simulink model "test_mdl_NI"  (R2018a)
settings: Solver=VariableStepAuto  StartTime=0.0  StopTime=10.0  RelTol=1e-3
(part 14 of 24)

== system test_mdl_NI/Subsystem/SOBDMC_HPCM_FD1/GoTimeSettings_FD1_Ox3F8 ==
  in_port : Inport
  ChrgGoTAllOn_B_Stat : Terminator
  ChrgGoTElement_B_Dsply : Terminator
  ChrgGoTElement_D_Stat : Terminator
  ChrgGoTExtHtrEnbl_B_Rq : Terminator
  ChrgGoTExtHtr_B_Stat : Terminator
  ChrgGoTHr_T_Stat : Terminator
  ChrgGoTMnte_D_Stat : Terminator
  ChrgGoTNext_D_Stat : Terminator
  ChrgGoTPrcond_D_Stat : Terminator
  ChrgGoTTouchEnbl_B_Rq : Terminator
  ChrgGoTTouch_B_Stat : Terminator
  ChrgLocIdCurnt_D_Uns : Terminator
  bus_selector : BusSelector  OutputSignals=ChrgGoTAllOn_B_Stat,ChrgGoTElement_B_Dsply,ChrgGoTElement_D_Stat,ChrgGoTExtHtrEnbl_B_Rq,ChrgGoTExtHtr_B_Stat,ChrgGoTHr_T_Stat,ChrgGoTMnte_D_Stat,ChrgGoTNext_D_Stat,ChrgGoTPrcond_D_Stat,ChrgGoTTouchEnbl_B_Rq,ChrgGoTTouch_B_Stat,ChrgLocIdCurnt_D_Uns
  wires:
  in_port/1 -> bus_selector/1  "GoTimeSettings_FD1_Ox3F8"
  bus_selector/1 -> ChrgGoTAllOn_B_Stat/1  "<ChrgGoTAllOn_B_Stat>"
  bus_selector/2 -> ChrgGoTElement_B_Dsply/1  "<ChrgGoTElement_B_Dsply>"
  bus_selector/3 -> ChrgGoTElement_D_Stat/1  "<ChrgGoTElement_D_Stat>"
  bus_selector/4 -> ChrgGoTExtHtrEnbl_B_Rq/1  "<ChrgGoTExtHtrEnbl_B_Rq>"
  bus_selector/5 -> ChrgGoTExtHtr_B_Stat/1  "<ChrgGoTExtHtr_B_Stat>"
  bus_selector/6 -> ChrgGoTHr_T_Stat/1  "<ChrgGoTHr_T_Stat>"
  bus_selector/7 -> ChrgGoTMnte_D_Stat/1  "<ChrgGoTMnte_D_Stat>"
  bus_selector/8 -> ChrgGoTNext_D_Stat/1  "<ChrgGoTNext_D_Stat>"
  bus_selector/9 -> ChrgGoTPrcond_D_Stat/1  "<ChrgGoTPrcond_D_Stat>"
  bus_selector/10 -> ChrgGoTTouchEnbl_B_Rq/1  "<ChrgGoTTouchEnbl_B_Rq>"
  bus_selector/11 -> ChrgGoTTouch_B_Stat/1  "<ChrgGoTTouch_B_Stat>"
  bus_selector/12 -> ChrgLocIdCurnt_D_Uns/1  "<ChrgLocIdCurnt_D_Uns>"

== system test_mdl_NI/Subsystem/SOBDMC_HPCM_FD1/HEV_ChargeStat_FD1_Ox352 ==
  in_port : Inport
  ChargeNowDuration_St : Terminator
  EstmChrgTimeHP_St : Terminator
  EstmChrgTimeLP_St : Terminator
  NxtUsgSocEst_Pc_Dsply : Terminator
  VehElRngeNut_L_Dsply : Terminator
  bus_selector : BusSelector  OutputSignals=ChargeNowDuration_St,EstmChrgTimeHP_St,EstmChrgTimeLP_St,NxtUsgSocEst_Pc_Dsply,VehElRngeNut_L_Dsply
  wires:
  in_port/1 -> bus_selector/1  "HEV_ChargeStat_FD1_Ox352"
  bus_selector/1 -> ChargeNowDuration_St/1  "<ChargeNowDuration_St>"
  bus_selector/2 -> EstmChrgTimeHP_St/1  "<EstmChrgTimeHP_St>"
  bus_selector/3 -> EstmChrgTimeLP_St/1  "<EstmChrgTimeLP_St>"
  bus_selector/4 -> NxtUsgSocEst_Pc_Dsply/1  "<NxtUsgSocEst_Pc_Dsply>"
  bus_selector/5 -> VehElRngeNut_L_Dsply/1  "<VehElRngeNut_L_Dsply>"

== system test_mdl_NI/Subsystem/SOBDMC_HPCM_FD1/MHT_EV_Wakeup_FD1_Ox478 ==
  in_port : Inport
  BattChlrSov_B_Rq : Terminator
  BattChrgTrgtSoC_D_Rq : Terminator
  BattTracClntVlv_B_Rq : Terminator
  BattTracDrvSustn_B_Rq : Terminator
  BrkAppl_D_RqPt : Terminator
  CabinDrvSustn_B_Rq : Terminator
  CabnEvapSovFront_B_Rq : Terminator
  CabnEvapSovRear_B_Rq : Terminator
  ChrgNowEvnt_B_Stat : Terminator
  HeatCoreSovRear_B_Rq : Terminator
  HtrnClntFlw_D_Rq : Terminator
  HtrnCnnctPwr_B_Stat : Terminator
  HtrnDcdcDis_B_Rq : Terminator
  PreCondBatt_B_Actl : Terminator
  PtcHtr_D_Stat : Terminator
  WakeAlarm0_B_Typ : Terminator
  WakeAlarm0_T_Rq : Terminator
  bus_selector : BusSelector  OutputSignals=BattChlrSov_B_Rq,BattChrgTrgtSoC_D_Rq,BattTracClntVlv_B_Rq,BattTracDrvSustn_B_Rq,BrkAppl_D_RqPt,CabinDrvSustn_B_Rq,CabnEvapSovFront_B_Rq,CabnEvapSovRear_B_Rq,ChrgNowEvnt_B_Stat,HeatCoreSovRear_B_Rq,HtrnClntFlw_D_Rq,HtrnCnnctPwr_B_Stat,HtrnDcdcDis_B_Rq,PreCondBatt_B_Actl,PtcHtr_D_Stat,WakeAlarm0_B_Typ,WakeAlarm0_T_Rq
  wires:
  in_port/1 -> bus_selector/1  "MHT_EV_Wakeup_FD1_Ox478"
  bus_selector/1 -> BattChlrSov_B_Rq/1  "<BattChlrSov_B_Rq>"
  bus_selector/2 -> BattChrgTrgtSoC_D_Rq/1  "<BattChrgTrgtSoC_D_Rq>"
  bus_selector/3 -> BattTracClntVlv_B_Rq/1  "<BattTracClntVlv_B_Rq>"
  bus_selector/4 -> BattTracDrvSustn_B_Rq/1  "<BattTracDrvSustn_B_Rq>"
  bus_selector/5 -> BrkAppl_D_RqPt/1  "<BrkAppl_D_RqPt>"
  bus_selector/6 -> CabinDrvSustn_B_Rq/1  "<CabinDrvSustn_B_Rq>"
  bus_selector/7 -> CabnEvapSovFront_B_Rq/1  "<CabnEvapSovFront_B_Rq>"
  bus_selector/8 -> CabnEvapSovRear_B_Rq/1  "<CabnEvapSovRear_B_Rq>"
  bus_selector/9 -> ChrgNowEvnt_B_Stat/1  "<ChrgNowEvnt_B_Stat>"
  bus_selector/10 -> HeatCoreSovRear_B_Rq/1  "<HeatCoreSovRear_B_Rq>"
  bus_selector/11 -> HtrnClntFlw_D_Rq/1  "<HtrnClntFlw_D_Rq>"
  bus_selector/12 -> HtrnCnnctPwr_B_Stat/1  "<HtrnCnnctPwr_B_Stat>"
  bus_selector/13 -> HtrnDcdcDis_B_Rq/1  "<HtrnDcdcDis_B_Rq>"
  bus_selector/14 -> PreCondBatt_B_Actl/1  "<PreCondBatt_B_Actl>"
  bus_selector/15 -> PtcHtr_D_Stat/1  "<PtcHtr_D_Stat>"
  bus_selector/16 -> WakeAlarm0_B_Typ/1  "<WakeAlarm0_B_Typ>"
  bus_selector/17 -> WakeAlarm0_T_Rq/1  "<WakeAlarm0_T_Rq>"

== system test_mdl_NI/Subsystem/SOBDMC_HPCM_FD1/MtrTracData_1_FD1_Ox441 ==
  in_port : Inport
  Inv1_Te_Actl : Terminator
  Mtr2Aout_W_ActlMntr : Terminator
  Mtr2CntlTeAlrm_B_Stat : Terminator
  MtrTrac2Coil_Te_Actl : Terminator
  MtrTrac2Falt_B_Stat : Terminator
  MtrTrac2Inv_Te_Actl : Terminator
  MtrTrac2TeAlrm_B_Stat : Terminator
  MtrTrac2_I_Actl : Terminator
  MtrTrac2_U_Actl : Terminator
  bus_selector : BusSelector  OutputSignals=Inv1_Te_Actl,Mtr2Aout_W_ActlMntr,Mtr2CntlTeAlrm_B_Stat,MtrTrac2Coil_Te_Actl,MtrTrac2Falt_B_Stat,MtrTrac2Inv_Te_Actl,MtrTrac2TeAlrm_B_Stat,MtrTrac2_I_Actl,MtrTrac2_U_Actl
  wires:
  in_port/1 -> bus_selector/1  "MtrTracData_1_FD1_Ox441"
  bus_selector/1 -> Inv1_Te_Actl/1  "<Inv1_Te_Actl>"
  bus_selector/2 -> Mtr2Aout_W_ActlMntr/1  "<Mtr2Aout_W_ActlMntr>"
  bus_selector/3 -> Mtr2CntlTeAlrm_B_Stat/1  "<Mtr2CntlTeAlrm_B_Stat>"
  bus_selector/4 -> MtrTrac2Coil_Te_Actl/1  "<MtrTrac2Coil_Te_Actl>"
  bus_selector/5 -> MtrTrac2Falt_B_Stat/1  "<MtrTrac2Falt_B_Stat>"
  bus_selector/6 -> MtrTrac2Inv_Te_Actl/1  "<MtrTrac2Inv_Te_Actl>"
  bus_selector/7 -> MtrTrac2TeAlrm_B_Stat/1  "<MtrTrac2TeAlrm_B_Stat>"
  bus_selector/8 -> MtrTrac2_I_Actl/1  "<MtrTrac2_I_Actl>"
  bus_selector/9 -> MtrTrac2_U_Actl/1  "<MtrTrac2_U_Actl>"

== system test_mdl_NI/Subsystem/SOBDMC_HPCM_FD1/MtrTrac_Data2_FD1_Ox442 ==
  in_port : Inport
  ChrgStat_D_ActlMntr : Terminator
  HybVehMde_D_ActlMntr : Terminator
  Inv1Ain_I_ActlMntr : Terminator
  Mtr2State_D_ActlMntr : Terminator
  VehElRnge_L_Dsply : Terminator
  bus_selector : BusSelector  OutputSignals=ChrgStat_D_ActlMntr,HybVehMde_D_ActlMntr,Inv1Ain_I_ActlMntr,Mtr2State_D_ActlMntr,VehElRnge_L_Dsply
  wires:
  in_port/1 -> bus_selector/1  "MtrTrac_Data2_FD1_Ox442"
  bus_selector/1 -> ChrgStat_D_ActlMntr/1  "<ChrgStat_D_ActlMntr>"
  bus_selector/2 -> HybVehMde_D_ActlMntr/1  "<HybVehMde_D_ActlMntr>"
  bus_selector/3 -> Inv1Ain_I_ActlMntr/1  "<Inv1Ain_I_ActlMntr>"
  bus_selector/4 -> Mtr2State_D_ActlMntr/1  "<Mtr2State_D_ActlMntr>"
  bus_selector/5 -> VehElRnge_L_Dsply/1  "<VehElRnge_L_Dsply>"

== system test_mdl_NI/Subsystem/SOBDMC_HPCM_FD1/OTAPhysSOBDMCtoGWM_FD1_Ox1B936011 ==
  in_port : Inport
  OTAPhysHPCMtoGWM_ECG : Terminator
  bus_selector : BusSelector  OutputSignals=OTAPhysHPCMtoGWM_ECG
  wires:
  in_port/1 -> bus_selector/1  "OTAPhysSOBDMCtoGWM_FD1_Ox1B936011"
  bus_selector/1 -> OTAPhysHPCMtoGWM_ECG/1  "<OTAPhysHPCMtoGWM_ECG>"

== system test_mdl_NI/Subsystem/SOBDMC_HPCM_FD1/PARSEDHPCMtoGWM_ECG_FD1_Ox1BA36011 ==
  in_port : Inport
  PARSEDPhysHPCMtoGWM_ECG : Terminator
  bus_selector : BusSelector  OutputSignals=PARSEDPhysHPCMtoGWM_ECG
  wires:
  in_port/1 -> bus_selector/1  "PARSEDHPCMtoGWM_ECG_FD1_Ox1BA36011"
  bus_selector/1 -> PARSEDPhysHPCMtoGWM_ECG/1  "<PARSEDPhysHPCMtoGWM_ECG>"

== system test_mdl_NI/Subsystem/SOBDMC_HPCM_FD1/PARSEDPushSOBDMCtoGWM_FD1_Ox1BB36011 ==
  in_port : Inport
  PARSEDPhysHPCM2toGWM_ECG : Terminator
  bus_selector : BusSelector  OutputSignals=PARSEDPhysHPCM2toGWM_ECG
  wires:
  in_port/1 -> bus_selector/1  "PARSEDPushSOBDMCtoGWM_FD1_Ox1BB36011"
  bus_selector/1 -> PARSEDPhysHPCM2toGWM_ECG/1  "<PARSEDPhysHPCM2toGWM_ECG>"

== system test_mdl_NI/Subsystem/SOBDMC_HPCM_FD1/PreCond_Hev_Data1_FD1_Ox440 ==
  in_port : Inport
  BattChrgInhbt_D_Rq : Terminator
  ChrgStat_D2_Dsply : Terminator
  ChrgTMatch_B_Stat : Terminator
  HvacPrecondAC_D_Rq : Terminator
  HvacPrecondBlwr2_D_Rq : Terminator
  HvacPrecondMode2_D_Rq : Terminator
  HvacPrecondRecirc_D_Rq : Terminator
  HvacPrecond_Te_Rq : Terminator
  bus_selector : BusSelector  OutputSignals=BattChrgInhbt_D_Rq,ChrgStat_D2_Dsply,ChrgTMatch_B_Stat,HvacPrecondAC_D_Rq,HvacPrecondBlwr2_D_Rq,HvacPrecondMode2_D_Rq,HvacPrecondRecirc_D_Rq,HvacPrecond_Te_Rq
  wires:
  in_port/1 -> bus_selector/1  "PreCond_Hev_Data1_FD1_Ox440"
  bus_selector/1 -> BattChrgInhbt_D_Rq/1  "<BattChrgInhbt_D_Rq>"
  bus_selector/2 -> ChrgStat_D2_Dsply/1  "<ChrgStat_D2_Dsply>"
  bus_selector/3 -> ChrgTMatch_B_Stat/1  "<ChrgTMatch_B_Stat>"
  bus_selector/4 -> HvacPrecondAC_D_Rq/1  "<HvacPrecondAC_D_Rq>"
  bus_selector/5 -> HvacPrecondBlwr2_D_Rq/1  "<HvacPrecondBlwr2_D_Rq>"
  bus_selector/6 -> HvacPrecondMode2_D_Rq/1  "<HvacPrecondMode2_D_Rq>"
  bus_selector/7 -> HvacPrecondRecirc_D_Rq/1  "<HvacPrecondRecirc_D_Rq>"
  bus_selector/8 -> HvacPrecond_Te_Rq/1  "<HvacPrecond_Te_Rq>"

== system test_mdl_NI/Subsystem/SOBDMC_HPCM_FD1/PreCond_Hev_Data2_FD1_Ox185 ==
  in_port : Inport
  BattTracClntFlw_Pc_Rq : Terminator
  BattTrac_I_EstVsc : Terminator
  DrvCondTpRrDefrs_B_Rq : Terminator
  HtrnAin_UHi_Actl : Terminator
  HtrnHvilOpen_B_Actl : Terminator
  HtrnMil_D_Rq : Terminator
  HtrnOvrTeLamp_B_Dsply : Terminator
  HtrnSrvcRqd_B_Dsply : Terminator
  PreCondActv_B_Actl : Terminator
  PtWakeupDeltaT_T_Rq : Terminator
  bus_selector : BusSelector  OutputSignals=BattTracClntFlw_Pc_Rq,BattTrac_I_EstVsc,DrvCondTpRrDefrs_B_Rq,HtrnAin_UHi_Actl,HtrnHvilOpen_B_Actl,HtrnMil_D_Rq,HtrnOvrTeLamp_B_Dsply,HtrnSrvcRqd_B_Dsply,PreCondActv_B_Actl,PtWakeupDeltaT_T_Rq
  wires:
  in_port/1 -> bus_selector/1  "PreCond_Hev_Data2_FD1_Ox185"
  bus_selector/1 -> BattTracClntFlw_Pc_Rq/1  "<BattTracClntFlw_Pc_Rq>"
  bus_selector/2 -> BattTrac_I_EstVsc/1  "<BattTrac_I_EstVsc>"
  bus_selector/3 -> DrvCondTpRrDefrs_B_Rq/1  "<DrvCondTpRrDefrs_B_Rq>"
  bus_selector/4 -> HtrnAin_UHi_Actl/1  "<HtrnAin_UHi_Actl>"
  bus_selector/5 -> HtrnHvilOpen_B_Actl/1  "<HtrnHvilOpen_B_Actl>"
  bus_selector/6 -> HtrnMil_D_Rq/1  "<HtrnMil_D_Rq>"
  bus_selector/7 -> HtrnOvrTeLamp_B_Dsply/1  "<HtrnOvrTeLamp_B_Dsply>"
  bus_selector/8 -> HtrnSrvcRqd_B_Dsply/1  "<HtrnSrvcRqd_B_Dsply>"
  bus_selector/9 -> PreCondActv_B_Actl/1  "<PreCondActv_B_Actl>"
  bus_selector/10 -> PtWakeupDeltaT_T_Rq/1  "<PtWakeupDeltaT_T_Rq>"

== system test_mdl_NI/Subsystem/SOBDMC_HPCM_FD1/SOBDMC_AutoSar_NetMgmt_FD1_Ox5A5 ==
  in_port : Inport
  SOBDMC_AutoSarNMControl : Terminator
  SOBDMC_AutoSarNMNodeId : Terminator
  SOBDMC_AutoSarNMReserved{1..4} (4 alike) : Terminator
  SOBDMC_GWNMProxy : Terminator
  SOBDMC_GWOnBoardTester : Terminator
  bus_selector : BusSelector  OutputSignals=SOBDMC_AutoSarNMControl,SOBDMC_AutoSarNMNodeId,SOBDMC_AutoSarNMReserved1,SOBDMC_AutoSarNMReserved2,SOBDMC_AutoSarNMReserved3,SOBDMC_AutoSarNMReserved4,SOBDMC_GWNMProxy,SOBDMC_GWOnBoardTester
  wires:
  in_port/1 -> bus_selector/1  "SOBDMC_AutoSar_NetMgmt_FD1_Ox5A5"
  bus_selector/1 -> SOBDMC_AutoSarNMControl/1  "<SOBDMC_AutoSarNMControl>"
  bus_selector/2 -> SOBDMC_AutoSarNMNodeId/1  "<SOBDMC_AutoSarNMNodeId>"
  bus_selector/3 -> SOBDMC_AutoSarNMReserved1/1  "<SOBDMC_AutoSarNMReserved1>"
  bus_selector/4 -> SOBDMC_AutoSarNMReserved2/1  "<SOBDMC_AutoSarNMReserved2>"
  bus_selector/5 -> SOBDMC_AutoSarNMReserved3/1  "<SOBDMC_AutoSarNMReserved3>"
  bus_selector/6 -> SOBDMC_AutoSarNMReserved4/1  "<SOBDMC_AutoSarNMReserved4>"
  bus_selector/7 -> SOBDMC_GWNMProxy/1  "<SOBDMC_GWNMProxy>"
  bus_selector/8 -> SOBDMC_GWOnBoardTester/1  "<SOBDMC_GWOnBoardTester>"

== system test_mdl_NI/Subsystem/SOBDMC_HPCM_FD1/SOBDMC_RapidData_Resp1_FD1_Ox68C ==
  in_port : Inport
  UUDTSOBDMCResponse1 : Terminator
  bus_selector : BusSelector  OutputSignals=UUDTSOBDMCResponse1
  wires:
  in_port/1 -> bus_selector/1  "SOBDMC_RapidData_Resp1_FD1_Ox68C"
  bus_selector/1 -> UUDTSOBDMCResponse1/1  "<UUDTSOBDMCResponse1>"

== system test_mdl_NI/Subsystem/SOBDMC_HPCM_FD1/SOBDMC_RapidData_Resp2_FD1_Ox68D ==
  in_port : Inport
  UUDTSOBDMCResponse2 : Terminator
  bus_selector : BusSelector  OutputSignals=UUDTSOBDMCResponse2
  wires:
  in_port/1 -> bus_selector/1  "SOBDMC_RapidData_Resp2_FD1_Ox68D"
  bus_selector/1 -> UUDTSOBDMCResponse2/1  "<UUDTSOBDMCResponse2>"

== system test_mdl_NI/Subsystem/SOBDMC_HPCM_FD1/SOBDMC_RapidData_Resp3_FD1_Ox68E ==
  in_port : Inport
  UUDTSOBDMCResponse3 : Terminator
  bus_selector : BusSelector  OutputSignals=UUDTSOBDMCResponse3
  wires:
  in_port/1 -> bus_selector/1  "SOBDMC_RapidData_Resp3_FD1_Ox68E"
  bus_selector/1 -> UUDTSOBDMCResponse3/1  "<UUDTSOBDMCResponse3>"

== system test_mdl_NI/Subsystem/SOBDMC_HPCM_FD1/SOBDMC_RapidData_Resp4_FD1_Ox68F ==
  in_port : Inport
  UUDTSOBDMCResponse4 : Terminator
  bus_selector : BusSelector  OutputSignals=UUDTSOBDMCResponse4
  wires:
  in_port/1 -> bus_selector/1  "SOBDMC_RapidData_Resp4_FD1_Ox68F"
  bus_selector/1 -> UUDTSOBDMCResponse4/1  "<UUDTSOBDMCResponse4>"

== system test_mdl_NI/Subsystem/SOBDMC_HPCM_FD1/Saved_Charge_Location_FD1_Ox3F4 ==
  in_port : Inport
  ChrgLocId_D_Sav : Terminator
  ChrgLocLattDeg_An_Sav : Terminator
  ChrgLocLattFrct_An_Sav : Terminator
  ChrgLocLattPostv_B_Sav : Terminator
  ChrgLocLongDeg_An_Sav : Terminator
  ChrgLocLongFrct_An_Sav : Terminator
  ChrgLocLongPostv_B_Sav : Terminator
  ChrgLocSaved_B_Dsply : Terminator
  ChrgNowCurnt_B_Dsply : Terminator
  bus_selector : BusSelector  OutputSignals=ChrgLocId_D_Sav,ChrgLocLattDeg_An_Sav,ChrgLocLattFrct_An_Sav,ChrgLocLattPostv_B_Sav,ChrgLocLongDeg_An_Sav,ChrgLocLongFrct_An_Sav,ChrgLocLongPostv_B_Sav,ChrgLocSaved_B_Dsply,ChrgNowCurnt_B_Dsply
  wires:
  in_port/1 -> bus_selector/1  "Saved_Charge_Location_FD1_Ox3F4"
  bus_selector/1 -> ChrgLocId_D_Sav/1  "<ChrgLocId_D_Sav>"
  bus_selector/2 -> ChrgLocLattDeg_An_Sav/1  "<ChrgLocLattDeg_An_Sav>"
  bus_selector/3 -> ChrgLocLattFrct_An_Sav/1  "<ChrgLocLattFrct_An_Sav>"
  bus_selector/4 -> ChrgLocLattPostv_B_Sav/1  "<ChrgLocLattPostv_B_Sav>"
  bus_selector/5 -> ChrgLocLongDeg_An_Sav/1  "<ChrgLocLongDeg_An_Sav>"
  bus_selector/6 -> ChrgLocLongFrct_An_Sav/1  "<ChrgLocLongFrct_An_Sav>"
  bus_selector/7 -> ChrgLocLongPostv_B_Sav/1  "<ChrgLocLongPostv_B_Sav>"
  bus_selector/8 -> ChrgLocSaved_B_Dsply/1  "<ChrgLocSaved_B_Dsply>"
  bus_selector/9 -> ChrgNowCurnt_B_Dsply/1  "<ChrgNowCurnt_B_Dsply>"

== system test_mdl_NI/Subsystem/SOBDMC_HPCM_FD1/TesterPhysicalResSOBDMCFD1_Ox7EE ==
  in_port : Inport
  TesterPhysicalResSOBDMC : Terminator
  bus_selector : BusSelector  OutputSignals=TesterPhysicalResSOBDMC
  wires:
  in_port/1 -> bus_selector/1  "TesterPhysicalResSOBDMCFD1_Ox7EE"
  bus_selector/1 -> TesterPhysicalResSOBDMC/1  "<TesterPhysicalResSOBDMC>"

== system test_mdl_NI/Subsystem/SOBDMC_HPCM_FD1/Unsaved_Charge_LocationFD1_Ox3F3 ==
  in_port : Inport
  ChrgLocId_D_Uns : Terminator
  ChrgLocLattDeg_An_Uns : Terminator
  ChrgLocLattFrct_An_Uns : Terminator
  ChrgLocLattPostv_B_Uns : Terminator
  ChrgLocLongDeg_An_Uns : Terminator
  ChrgLocLongFrct_An_Uns : Terminator
  ChrgLocLongPostv_B_Uns : Terminator
  bus_selector : BusSelector  OutputSignals=ChrgLocId_D_Uns,ChrgLocLattDeg_An_Uns,ChrgLocLattFrct_An_Uns,ChrgLocLattPostv_B_Uns,ChrgLocLongDeg_An_Uns,ChrgLocLongFrct_An_Uns,ChrgLocLongPostv_B_Uns
  wires:
  in_port/1 -> bus_selector/1  "Unsaved_Charge_LocationFD1_Ox3F3"
  bus_selector/1 -> ChrgLocId_D_Uns/1  "<ChrgLocId_D_Uns>"
  bus_selector/2 -> ChrgLocLattDeg_An_Uns/1  "<ChrgLocLattDeg_An_Uns>"
  bus_selector/3 -> ChrgLocLattFrct_An_Uns/1  "<ChrgLocLattFrct_An_Uns>"
  bus_selector/4 -> ChrgLocLattPostv_B_Uns/1  "<ChrgLocLattPostv_B_Uns>"
  bus_selector/5 -> ChrgLocLongDeg_An_Uns/1  "<ChrgLocLongDeg_An_Uns>"
  bus_selector/6 -> ChrgLocLongFrct_An_Uns/1  "<ChrgLocLongFrct_An_Uns>"
  bus_selector/7 -> ChrgLocLongPostv_B_Uns/1  "<ChrgLocLongPostv_B_Uns>"

== system test_mdl_NI/Subsystem/TCCM/AWD_Torque_Data_Ox20C ==
  in_port : Inport
  PrplWhlTotTqRqMxAwd_No_Cnt : Terminator
  PrplWhlTotTqRqMxAwd_No_Cs : Terminator
  PrplWhlTot_Tq_RqMxAwd : Terminator
  bus_selector : BusSelector  OutputSignals=PrplWhlTotTqRqMxAwd_No_Cnt,PrplWhlTotTqRqMxAwd_No_Cs,PrplWhlTot_Tq_RqMxAwd
  wires:
  in_port/1 -> bus_selector/1  "AWD_Torque_Data_Ox20C"
  bus_selector/1 -> PrplWhlTotTqRqMxAwd_No_Cnt/1  "<PrplWhlTotTqRqMxAwd_No_Cnt>"
  bus_selector/2 -> PrplWhlTotTqRqMxAwd_No_Cs/1  "<PrplWhlTotTqRqMxAwd_No_Cs>"
  bus_selector/3 -> PrplWhlTot_Tq_RqMxAwd/1  "<PrplWhlTot_Tq_RqMxAwd>"

== system test_mdl_NI/Subsystem/TCCM/Driveline_Data_1_Ox263 ==
  in_port : Inport
  Awd2wdLamp_D_RqDsply : Terminator
  AwdAutoLamp_D_RqDsply : Terminator
  AwdHiLamp_D_RqDsply : Terminator
  AwdLck_D_Stat : Terminator
  AwdLck_Tq_Rq : Terminator
  AwdLoLamp_D_RqDsply : Terminator
  AwdOffRoadMode_D_Stats : Terminator
  AwdRnge_D_Actl : Terminator
  AwdSrvcRqd_B_Rq : Terminator
  AwdStat_D_RqDsply : Terminator
  AwdSys_D_Stat : Terminator
  NtrlTowAvail_B_Stat : Terminator
  TrnAout_Tq_RqMx : Terminator
  bus_selector : BusSelector  OutputSignals=Awd2wdLamp_D_RqDsply,AwdAutoLamp_D_RqDsply,AwdHiLamp_D_RqDsply,AwdLck_D_Stat,AwdLck_Tq_Rq,AwdLoLamp_D_RqDsply,AwdOffRoadMode_D_Stats,AwdRnge_D_Actl,AwdSrvcRqd_B_Rq,AwdStat_D_RqDsply,AwdSys_D_Stat,NtrlTowAvail_B_Stat,TrnAout_Tq_RqMx
  wires:
  in_port/1 -> bus_selector/1  "Driveline_Data_1_Ox263"
  bus_selector/1 -> Awd2wdLamp_D_RqDsply/1  "<Awd2wdLamp_D_RqDsply>"
  bus_selector/2 -> AwdAutoLamp_D_RqDsply/1  "<AwdAutoLamp_D_RqDsply>"
  bus_selector/3 -> AwdHiLamp_D_RqDsply/1  "<AwdHiLamp_D_RqDsply>"
  bus_selector/4 -> AwdLck_D_Stat/1  "<AwdLck_D_Stat>"
  bus_selector/5 -> AwdLck_Tq_Rq/1  "<AwdLck_Tq_Rq>"
  bus_selector/6 -> AwdLoLamp_D_RqDsply/1  "<AwdLoLamp_D_RqDsply>"
  bus_selector/7 -> AwdOffRoadMode_D_Stats/1  "<AwdOffRoadMode_D_Stats>"
  bus_selector/8 -> AwdRnge_D_Actl/1  "<AwdRnge_D_Actl>"
  bus_selector/9 -> AwdSrvcRqd_B_Rq/1  "<AwdSrvcRqd_B_Rq>"
  bus_selector/10 -> AwdStat_D_RqDsply/1  "<AwdStat_D_RqDsply>"
  bus_selector/11 -> AwdSys_D_Stat/1  "<AwdSys_D_Stat>"
  bus_selector/12 -> NtrlTowAvail_B_Stat/1  "<NtrlTowAvail_B_Stat>"
  bus_selector/13 -> TrnAout_Tq_RqMx/1  "<TrnAout_Tq_RqMx>"

== system test_mdl_NI/Subsystem/TCCM/Driveline_Data_2_Ox4A2 ==
  in_port : Inport
  LsdSrvcRqd_B_Rq : Terminator
  RearDiffFalt_D_Stat : Terminator
  RearDiffLckLamp_D_Rq : Terminator
  RearDiffLckMsg_D_Rq : Terminator
  RearDiffLck_Tq_Actl : Terminator
  SelDrvMdeAwd2_D_Stat : Terminator
  bus_selector : BusSelector  OutputSignals=LsdSrvcRqd_B_Rq,RearDiffFalt_D_Stat,RearDiffLckLamp_D_Rq,RearDiffLckMsg_D_Rq,RearDiffLck_Tq_Actl,SelDrvMdeAwd2_D_Stat
  wires:
  in_port/1 -> bus_selector/1  "Driveline_Data_2_Ox4A2"
  bus_selector/1 -> LsdSrvcRqd_B_Rq/1  "<LsdSrvcRqd_B_Rq>"
  bus_selector/2 -> RearDiffFalt_D_Stat/1  "<RearDiffFalt_D_Stat>"
  bus_selector/3 -> RearDiffLckLamp_D_Rq/1  "<RearDiffLckLamp_D_Rq>"
  bus_selector/4 -> RearDiffLckMsg_D_Rq/1  "<RearDiffLckMsg_D_Rq>"
  bus_selector/5 -> RearDiffLck_Tq_Actl/1  "<RearDiffLck_Tq_Actl>"
  bus_selector/6 -> SelDrvMdeAwd2_D_Stat/1  "<SelDrvMdeAwd2_D_Stat>"

== system test_mdl_NI/Subsystem/TCCM/TCCM_AutoSar_NetwkMgmt_Ox5A1 ==
  in_port : Inport
  TCCM_AutoSarNMControl : Terminator
  TCCM_AutoSarNMNodeId : Terminator
  TCCM_AutoSarNMReserved{1..4} (4 alike) : Terminator
  TCCM_GWNMProxy : Terminator
  TCCM_GWOnBoardTester : Terminator
  bus_selector : BusSelector  OutputSignals=TCCM_AutoSarNMControl,TCCM_AutoSarNMNodeId,TCCM_AutoSarNMReserved1,TCCM_AutoSarNMReserved2,TCCM_AutoSarNMReserved3,TCCM_AutoSarNMReserved4,TCCM_GWNMProxy,TCCM_GWOnBoardTester
  wires:
  in_port/1 -> bus_selector/1  "TCCM_AutoSar_NetwkMgmt_Ox5A1"
  bus_selector/1 -> TCCM_AutoSarNMControl/1  "<TCCM_AutoSarNMControl>"
  bus_selector/2 -> TCCM_AutoSarNMNodeId/1  "<TCCM_AutoSarNMNodeId>"
  bus_selector/3 -> TCCM_AutoSarNMReserved1/1  "<TCCM_AutoSarNMReserved1>"
  bus_selector/4 -> TCCM_AutoSarNMReserved2/1  "<TCCM_AutoSarNMReserved2>"
  bus_selector/5 -> TCCM_AutoSarNMReserved3/1  "<TCCM_AutoSarNMReserved3>"
  bus_selector/6 -> TCCM_AutoSarNMReserved4/1  "<TCCM_AutoSarNMReserved4>"
  bus_selector/7 -> TCCM_GWNMProxy/1  "<TCCM_GWNMProxy>"
  bus_selector/8 -> TCCM_GWOnBoardTester/1  "<TCCM_GWOnBoardTester>"

== system test_mdl_NI/Subsystem/TCCM/TesterPhysicalResTCCM_Ox769 ==
  in_port : Inport
  TesterPhysicalResTCCM : Terminator
  bus_selector : BusSelector  OutputSignals=TesterPhysicalResTCCM
  wires:
  in_port/1 -> bus_selector/1  "TesterPhysicalResTCCM_Ox769"
  bus_selector/1 -> TesterPhysicalResTCCM/1  "<TesterPhysicalResTCCM>"

== system test_mdl_NI/Subsystem/TCM_DSL/EngineData_1_Ox171 ==
  in_port : Inport
  SeatWorkSrfc_B_Falt : Terminator
  TrnIpcDsplyGear_D_Actl : Terminator
  TrnIpcDsplyGear_D_Stat : Terminator
  TrnIpcDsplyMde_D_Actl : Terminator
  TrnIpcDsplyMde_D_Stat : Terminator
  TrnIpcDsplyRng2_D_Actl : Terminator
  TrnIpcDsplyRng_D_Stat : Terminator
  bus_selector : BusSelector  OutputSignals=SeatWorkSrfc_B_Falt,TrnIpcDsplyGear_D_Actl,TrnIpcDsplyGear_D_Stat,TrnIpcDsplyMde_D_Actl,TrnIpcDsplyMde_D_Stat,TrnIpcDsplyRng2_D_Actl,TrnIpcDsplyRng_D_Stat
  wires:
  in_port/1 -> bus_selector/1  "EngineData_1_Ox171"
  bus_selector/1 -> SeatWorkSrfc_B_Falt/1  "<SeatWorkSrfc_B_Falt>"
  bus_selector/2 -> TrnIpcDsplyGear_D_Actl/1  "<TrnIpcDsplyGear_D_Actl>"
  bus_selector/3 -> TrnIpcDsplyGear_D_Stat/1  "<TrnIpcDsplyGear_D_Stat>"
  bus_selector/4 -> TrnIpcDsplyMde_D_Actl/1  "<TrnIpcDsplyMde_D_Actl>"
  bus_selector/5 -> TrnIpcDsplyMde_D_Stat/1  "<TrnIpcDsplyMde_D_Stat>"
  bus_selector/6 -> TrnIpcDsplyRng2_D_Actl/1  "<TrnIpcDsplyRng2_D_Actl>"
  bus_selector/7 -> TrnIpcDsplyRng_D_Stat/1  "<TrnIpcDsplyRng_D_Stat>"

== system test_mdl_NI/Subsystem/TCM_DSL/Gear_Shift_by_Wire_3_Ox5C ==
  in_port : Inport
  GearSelLck_D_Rq : Terminator
  PrkBrkActv_D_RqTrnGear : Terminator
  TrnCmdCnt_B_Actl : Terminator
  TrnCmdState_B_Actl : Terminator
  TrnDtpCmd_D_Actl : Terminator
  TrnGearCmd_No_Cnt : Terminator
  TrnGearCmd_No_Cs : Terminator
  TrnGearCmd_Pc_ActlPt : Terminator
  TrnGearMsgTxt_D_Rq : Terminator
  TrnGearNtmAllow_B_Stat : Terminator
  TrnGear_D_RqPt : Terminator
  TrnLvrV_D_Rq : Terminator
  TrnNtrlTowCmd_D_Actl : Terminator
  TrnSbwSysHlth_D_Actl : Terminator
  TrnValidGear_D_Cnfm : Terminator
  bus_selector : BusSelector  OutputSignals=GearSelLck_D_Rq,PrkBrkActv_D_RqTrnGear,TrnCmdCnt_B_Actl,TrnCmdState_B_Actl,TrnDtpCmd_D_Actl,TrnGearCmd_No_Cnt,TrnGearCmd_No_Cs,TrnGearCmd_Pc_ActlPt,TrnGearMsgTxt_D_Rq,TrnGearNtmAllow_B_Stat,TrnGear_D_RqPt,TrnLvrV_D_Rq,TrnNtrlTowCmd_D_Actl,TrnSbwSysHlth_D_Actl,TrnValidGear_D_Cnfm
  wires:
  in_port/1 -> bus_selector/1  "Gear_Shift_by_Wire_3_Ox5C"
  bus_selector/1 -> GearSelLck_D_Rq/1  "<GearSelLck_D_Rq>"
  bus_selector/2 -> PrkBrkActv_D_RqTrnGear/1  "<PrkBrkActv_D_RqTrnGear>"
  bus_selector/3 -> TrnCmdCnt_B_Actl/1  "<TrnCmdCnt_B_Actl>"
  bus_selector/4 -> TrnCmdState_B_Actl/1  "<TrnCmdState_B_Actl>"
  bus_selector/5 -> TrnDtpCmd_D_Actl/1  "<TrnDtpCmd_D_Actl>"
  bus_selector/6 -> TrnGearCmd_No_Cnt/1  "<TrnGearCmd_No_Cnt>"
  bus_selector/7 -> TrnGearCmd_No_Cs/1  "<TrnGearCmd_No_Cs>"
  bus_selector/8 -> TrnGearCmd_Pc_ActlPt/1  "<TrnGearCmd_Pc_ActlPt>"
  bus_selector/9 -> TrnGearMsgTxt_D_Rq/1  "<TrnGearMsgTxt_D_Rq>"
  bus_selector/10 -> TrnGearNtmAllow_B_Stat/1  "<TrnGearNtmAllow_B_Stat>"
  bus_selector/11 -> TrnGear_D_RqPt/1  "<TrnGear_D_RqPt>"
  bus_selector/12 -> TrnLvrV_D_Rq/1  "<TrnLvrV_D_Rq>"
  bus_selector/13 -> TrnNtrlTowCmd_D_Actl/1  "<TrnNtrlTowCmd_D_Actl>"
  bus_selector/14 -> TrnSbwSysHlth_D_Actl/1  "<TrnSbwSysHlth_D_Actl>"
  bus_selector/15 -> TrnValidGear_D_Cnfm/1  "<TrnValidGear_D_Cnfm>"

== system test_mdl_NI/Subsystem/TCM_DSL/PowertrainData_10_Ox176 ==
  in_port : Inport
  GearEngag_D_Actl : Terminator
  GearLvr_D_ActlDrv : Terminator
  GearPos_D_Actl : Terminator
  GearPos_D_Trg : Terminator
  GearPos_No_Cnt : Terminator
  GearPos_No_Cs : Terminator
  TrnIgnOffDly_T_Rq : Terminator
  TrnPrkSys_D_Actl : Terminator
  TrnRng_D_Rq : Terminator
  bus_selector : BusSelector  OutputSignals=GearEngag_D_Actl,GearLvr_D_ActlDrv,GearPos_D_Actl,GearPos_D_Trg,GearPos_No_Cnt,GearPos_No_Cs,TrnIgnOffDly_T_Rq,TrnPrkSys_D_Actl,TrnRng_D_Rq
  wires:
  in_port/1 -> bus_selector/1  "PowertrainData_10_Ox176"
  bus_selector/1 -> GearEngag_D_Actl/1  "<GearEngag_D_Actl>"
  bus_selector/2 -> GearLvr_D_ActlDrv/1  "<GearLvr_D_ActlDrv>"
  bus_selector/3 -> GearPos_D_Actl/1  "<GearPos_D_Actl>"
  bus_selector/4 -> GearPos_D_Trg/1  "<GearPos_D_Trg>"
  bus_selector/5 -> GearPos_No_Cnt/1  "<GearPos_No_Cnt>"
  bus_selector/6 -> GearPos_No_Cs/1  "<GearPos_No_Cs>"
  bus_selector/7 -> TrnIgnOffDly_T_Rq/1  "<TrnIgnOffDly_T_Rq>"
  bus_selector/8 -> TrnPrkSys_D_Actl/1  "<TrnPrkSys_D_Actl>"
  bus_selector/9 -> TrnRng_D_Rq/1  "<TrnRng_D_Rq>"

== system test_mdl_NI/Subsystem/TCM_DSL/TCM_AutoSar_NetworkMgt_Ox5A0 ==
  in_port : Inport
  TCM_AutoSarNMControl : Terminator
  TCM_AutoSarNMNodeId : Terminator
  TCM_AutoSarNMReserved{1..4} (4 alike) : Terminator
  TCM_GWNMProxy : Terminator
  TCM_GWOnBoardTester : Terminator
  bus_selector : BusSelector  OutputSignals=TCM_AutoSarNMControl,TCM_AutoSarNMNodeId,TCM_AutoSarNMReserved1,TCM_AutoSarNMReserved2,TCM_AutoSarNMReserved3,TCM_AutoSarNMReserved4,TCM_GWNMProxy,TCM_GWOnBoardTester
  wires:
  in_port/1 -> bus_selector/1  "TCM_AutoSar_NetworkMgt_Ox5A0"
  bus_selector/1 -> TCM_AutoSarNMControl/1  "<TCM_AutoSarNMControl>"
  bus_selector/2 -> TCM_AutoSarNMNodeId/1  "<TCM_AutoSarNMNodeId>"
  bus_selector/3 -> TCM_AutoSarNMReserved1/1  "<TCM_AutoSarNMReserved1>"
  bus_selector/4 -> TCM_AutoSarNMReserved2/1  "<TCM_AutoSarNMReserved2>"
  bus_selector/5 -> TCM_AutoSarNMReserved3/1  "<TCM_AutoSarNMReserved3>"
  bus_selector/6 -> TCM_AutoSarNMReserved4/1  "<TCM_AutoSarNMReserved4>"
  bus_selector/7 -> TCM_GWNMProxy/1  "<TCM_GWNMProxy>"
  bus_selector/8 -> TCM_GWOnBoardTester/1  "<TCM_GWOnBoardTester>"

== system test_mdl_NI/Subsystem/TCM_DSL/TCM_Rapid_Data_Response_1_Ox6A4 ==
  in_port : Inport
  UUDTTCMResponse1 : Terminator
  bus_selector : BusSelector  OutputSignals=UUDTTCMResponse1
  wires:
  in_port/1 -> bus_selector/1  "TCM_Rapid_Data_Response_1_Ox6A4"
  bus_selector/1 -> UUDTTCMResponse1/1  "<UUDTTCMResponse1>"

== system test_mdl_NI/Subsystem/TCM_DSL/TCM_Rapid_Data_Response_2_Ox6A5 ==
  in_port : Inport
  UUDTTCMResponse2 : Terminator
  bus_selector : BusSelector  OutputSignals=UUDTTCMResponse2
  wires:
  in_port/1 -> bus_selector/1  "TCM_Rapid_Data_Response_2_Ox6A5"
  bus_selector/1 -> UUDTTCMResponse2/1  "<UUDTTCMResponse2>"

== system test_mdl_NI/Subsystem/TCM_DSL/TesterPhysicalResTCM_Ox7E9 ==
  in_port : Inport
  TesterPhysicalResTCM : Terminator
  bus_selector : BusSelector  OutputSignals=TesterPhysicalResTCM
  wires:
  in_port/1 -> bus_selector/1  "TesterPhysicalResTCM_Ox7E9"
  bus_selector/1 -> TesterPhysicalResTCM/1  "<TesterPhysicalResTCM>"

== system test_mdl_NI/Subsystem/TCM_DSL/TransData_3_Ox14A ==
  in_port : Inport
  TrnAout_W_ActlUnfilt : Terminator
  bus_selector : BusSelector  OutputSignals=TrnAout_W_ActlUnfilt
  wires:
  in_port/1 -> bus_selector/1  "TransData_3_Ox14A"
  bus_selector/1 -> TrnAout_W_ActlUnfilt/1  "<TrnAout_W_ActlUnfilt>"

== system test_mdl_NI/Subsystem/TCM_DSL/TransGearData_2_Ox231 ==
  in_port : Inport
  TrnMsgTxt2_D_Rq : Terminator
  TrnMsgTxt_D_Rq : Terminator
  bus_selector : BusSelector  OutputSignals=TrnMsgTxt2_D_Rq,TrnMsgTxt_D_Rq
  wires:
  in_port/1 -> bus_selector/1  "TransGearData_2_Ox231"
  bus_selector/1 -> TrnMsgTxt2_D_Rq/1  "<TrnMsgTxt2_D_Rq>"
  bus_selector/2 -> TrnMsgTxt_D_Rq/1  "<TrnMsgTxt_D_Rq>"

== system test_mdl_NI/Subsystem/TCM_DSL/TransGearData_Ox230 ==
  in_port : Inport
  GboxOil_Te_Actl : Terminator
  GearLvrPos_D_Actl : Terminator
  SelDrvMdeSwtch_D_Stat3 : Terminator
  TrnShifActv_B_Actl : Terminator
  TrnSrvcRqd_B_Rq : Terminator
  bus_selector : BusSelector  OutputSignals=GboxOil_Te_Actl,GearLvrPos_D_Actl,SelDrvMdeSwtch_D_Stat3,TrnShifActv_B_Actl,TrnSrvcRqd_B_Rq
  wires:
  in_port/1 -> bus_selector/1  "TransGearData_Ox230"
  bus_selector/1 -> GboxOil_Te_Actl/1  "<GboxOil_Te_Actl>"
  bus_selector/2 -> GearLvrPos_D_Actl/1  "<GearLvrPos_D_Actl>"
  bus_selector/3 -> SelDrvMdeSwtch_D_Stat3/1  "<SelDrvMdeSwtch_D_Stat3>"
  bus_selector/4 -> TrnShifActv_B_Actl/1  "<TrnShifActv_B_Actl>"
  bus_selector/5 -> TrnSrvcRqd_B_Rq/1  "<TrnSrvcRqd_B_Rq>"

== system test_mdl_NI/Subsystem/TSTR/TesterFunctionalReq_FD1_Ox7DF ==
  in_port : Inport
  TesterFunctionalReq : Terminator
  bus_selector : BusSelector  OutputSignals=TesterFunctionalReq
  wires:
  in_port/1 -> bus_selector/1  "TesterFunctionalReq_FD1_Ox7DF"
  bus_selector/1 -> TesterFunctionalReq/1  "<TesterFunctionalReq>"

== system test_mdl_NI/Subsystem/TSTR/TesterPhysicalReqABS_Ox760 ==
  in_port : Inport
  TesterPhysicalReqABS : Terminator
  bus_selector : BusSelector  OutputSignals=TesterPhysicalReqABS
  wires:
  in_port/1 -> bus_selector/1  "TesterPhysicalReqABS_Ox760"
  bus_selector/1 -> TesterPhysicalReqABS/1  "<TesterPhysicalReqABS>"

== system test_mdl_NI/Subsystem/TSTR/TesterPhysicalReqCCM_Ox764 ==
  in_port : Inport
  TesterPhysicalReqCCM : Terminator
  bus_selector : BusSelector  OutputSignals=TesterPhysicalReqCCM
  wires:
  in_port/1 -> bus_selector/1  "TesterPhysicalReqCCM_Ox764"
  bus_selector/1 -> TesterPhysicalReqCCM/1  "<TesterPhysicalReqCCM>"

== system test_mdl_NI/Subsystem/TSTR/TesterPhysicalReqCMR_DSMC_Ox7C1 ==
  in_port : Inport
  TesterPhysicalReqCMR_DSMC : Terminator
  bus_selector : BusSelector  OutputSignals=TesterPhysicalReqCMR_DSMC
  wires:
  in_port/1 -> bus_selector/1  "TesterPhysicalReqCMR_DSMC_Ox7C1"
  bus_selector/1 -> TesterPhysicalReqCMR_DSMC/1  "<TesterPhysicalReqCMR_DSMC>"

== system test_mdl_NI/Subsystem/TSTR/TesterPhysicalReqGWM_FD1_Ox716 ==
  in_port : Inport
  TesterPhysicalReqGWM_F1 : Terminator
  bus_selector : BusSelector  OutputSignals=TesterPhysicalReqGWM_F1
  wires:
  in_port/1 -> bus_selector/1  "TesterPhysicalReqGWM_FD1_Ox716"
  bus_selector/1 -> TesterPhysicalReqGWM_F1/1  "<TesterPhysicalReqGWM_F1>"

== system test_mdl_NI/Subsystem/TSTR/TesterPhysicalReqIPMA_Ox706 ==
  in_port : Inport
  TesterPhysicalReqIPMA : Terminator
  bus_selector : BusSelector  OutputSignals=TesterPhysicalReqIPMA
  wires:
  in_port/1 -> bus_selector/1  "TesterPhysicalReqIPMA_Ox706"
  bus_selector/1 -> TesterPhysicalReqIPMA/1  "<TesterPhysicalReqIPMA>"

== system test_mdl_NI/Subsystem/TSTR/TesterPhysicalReqPCM_Ox7E0 ==
  in_port : Inport
  TesterPhysicalReqPCM : Terminator
  bus_selector : BusSelector  OutputSignals=TesterPhysicalReqPCM
  wires:
  in_port/1 -> bus_selector/1  "TesterPhysicalReqPCM_Ox7E0"
  bus_selector/1 -> TesterPhysicalReqPCM/1  "<TesterPhysicalReqPCM>"

== system test_mdl_NI/Subsystem/TSTR/TesterPhysicalReqPSCM_Ox730 ==
  in_port : Inport
  TesterPhysicalReqPSCM : Terminator
  bus_selector : BusSelector  OutputSignals=TesterPhysicalReqPSCM
  wires:
  in_port/1 -> bus_selector/1  "TesterPhysicalReqPSCM_Ox730"
  bus_selector/1 -> TesterPhysicalReqPSCM/1  "<TesterPhysicalReqPSCM>"

== system test_mdl_NI/Subsystem/TSTR/TesterPhysicalReqSOBDMC_FD_Ox7E6 ==
  in_port : Inport
  TesterPhysicalReqSOBDMC : Terminator
  bus_selector : BusSelector  OutputSignals=TesterPhysicalReqSOBDMC
  wires:
  in_port/1 -> bus_selector/1  "TesterPhysicalReqSOBDMC_FD_Ox7E6"
  bus_selector/1 -> TesterPhysicalReqSOBDMC/1  "<TesterPhysicalReqSOBDMC>"

== system test_mdl_NI/Subsystem/TSTR/TesterPhysicalReqSODCMC_Ox6F2 ==
  in_port : Inport
  TesterPhysicalReqSODCMC : Terminator
  bus_selector : BusSelector  OutputSignals=TesterPhysicalReqSODCMC
  wires:
  in_port/1 -> bus_selector/1  "TesterPhysicalReqSODCMC_Ox6F2"
  bus_selector/1 -> TesterPhysicalReqSODCMC/1  "<TesterPhysicalReqSODCMC>"

== system test_mdl_NI/Subsystem/TSTR/TesterPhysicalReqSODCMD_Ox6F3 ==
  in_port : Inport
  TesterPhysicalReqSODCMD : Terminator
  bus_selector : BusSelector  OutputSignals=TesterPhysicalReqSODCMD
  wires:
  in_port/1 -> bus_selector/1  "TesterPhysicalReqSODCMD_Ox6F3"
  bus_selector/1 -> TesterPhysicalReqSODCMD/1  "<TesterPhysicalReqSODCMD>"

== system test_mdl_NI/Subsystem/TSTR/TesterPhysicalReqSODL_Ox7C4 ==
  in_port : Inport
  TesterPhysicalReqSODL : Terminator
  bus_selector : BusSelector  OutputSignals=TesterPhysicalReqSODL
  wires:
  in_port/1 -> bus_selector/1  "TesterPhysicalReqSODL_Ox7C4"
  bus_selector/1 -> TesterPhysicalReqSODL/1  "<TesterPhysicalReqSODL>"

== system test_mdl_NI/Subsystem/TSTR/TesterPhysicalReqSODR_Ox7C6 ==
  in_port : Inport
  TesterPhysicalReqSODR : Terminator
  bus_selector : BusSelector  OutputSignals=TesterPhysicalReqSODR
  wires:
  in_port/1 -> bus_selector/1  "TesterPhysicalReqSODR_Ox7C6"
  bus_selector/1 -> TesterPhysicalReqSODR/1  "<TesterPhysicalReqSODR>"

== system test_mdl_NI/Subsystem/TSTR/TesterPhysicalReqTCCM_Ox761 ==
  in_port : Inport
  TesterPhysicalReqTCCM : Terminator
  bus_selector : BusSelector  OutputSignals=TesterPhysicalReqTCCM
  wires:
  in_port/1 -> bus_selector/1  "TesterPhysicalReqTCCM_Ox761"
  bus_selector/1 -> TesterPhysicalReqTCCM/1  "<TesterPhysicalReqTCCM>"

== system test_mdl_NI/Subsystem/TSTR/TesterPhysicalReqTCM_Ox7E1 ==
  in_port : Inport
  TesterPhysicalReqTCM : Terminator
  bus_selector : BusSelector  OutputSignals=TesterPhysicalReqTCM
  wires:
  in_port/1 -> bus_selector/1  "TesterPhysicalReqTCM_Ox7E1"
  bus_selector/1 -> TesterPhysicalReqTCM/1  "<TesterPhysicalReqTCM>"

== system test_mdl_NI/Subsystem/VDM/Suspension_Data_Ox23A ==
  in_port : Inport
  SuspClkSync_No_Rq : Terminator
  SuspFrntRight_L_Actl : Terminator
  SuspFrnt_L_Actl : Terminator
  SuspFrnt_L_Prev : Terminator
  SuspRearRight_L_Actl : Terminator
  SuspRear_L_Actl : Terminator
  SuspRear_L_Prev : Terminator
  bus_selector : BusSelector  OutputSignals=SuspClkSync_No_Rq,SuspFrntRight_L_Actl,SuspFrnt_L_Actl,SuspFrnt_L_Prev,SuspRearRight_L_Actl,SuspRear_L_Actl,SuspRear_L_Prev
  wires:
  in_port/1 -> bus_selector/1  "Suspension_Data_Ox23A"
  bus_selector/1 -> SuspClkSync_No_Rq/1  "<SuspClkSync_No_Rq>"
  bus_selector/2 -> SuspFrntRight_L_Actl/1  "<SuspFrntRight_L_Actl>"
  bus_selector/3 -> SuspFrnt_L_Actl/1  "<SuspFrnt_L_Actl>"
  bus_selector/4 -> SuspFrnt_L_Prev/1  "<SuspFrnt_L_Prev>"
  bus_selector/5 -> SuspRearRight_L_Actl/1  "<SuspRearRight_L_Actl>"
  bus_selector/6 -> SuspRear_L_Actl/1  "<SuspRear_L_Actl>"
  bus_selector/7 -> SuspRear_L_Prev/1  "<SuspRear_L_Prev>"

== system test_mdl_NI/Subsystem/VDM/TesterPhysicalResVDM_Ox729 ==
  in_port : Inport
  TesterPhysicalResVDM : Terminator
  bus_selector : BusSelector  OutputSignals=TesterPhysicalResVDM
  wires:
  in_port/1 -> bus_selector/1  "TesterPhysicalResVDM_Ox729"
  bus_selector/1 -> TesterPhysicalResVDM/1  "<TesterPhysicalResVDM>"

== system test_mdl_NI/Subsystem/VDM/VeyDynamics_Data_Ox345 ==
  in_port : Inport
  AdptDrvMdeChassis_D_Rq : Terminator
  AdptDrvMdePt_D_Rq : Terminator
  CcdMsgTxt_D_RqDsply : Terminator
  Ccd_B_Falt : Terminator
  SelDrvMdeSusp_D_Stat : Terminator
  bus_selector : BusSelector  OutputSignals=AdptDrvMdeChassis_D_Rq,AdptDrvMdePt_D_Rq,CcdMsgTxt_D_RqDsply,Ccd_B_Falt,SelDrvMdeSusp_D_Stat
  wires:
  in_port/1 -> bus_selector/1  "VeyDynamics_Data_Ox345"
  bus_selector/1 -> AdptDrvMdeChassis_D_Rq/1  "<AdptDrvMdeChassis_D_Rq>"
  bus_selector/2 -> AdptDrvMdePt_D_Rq/1  "<AdptDrvMdePt_D_Rq>"
  bus_selector/3 -> CcdMsgTxt_D_RqDsply/1  "<CcdMsgTxt_D_RqDsply>"
  bus_selector/4 -> Ccd_B_Falt/1  "<Ccd_B_Falt>"
  bus_selector/5 -> SelDrvMdeSusp_D_Stat/1  "<SelDrvMdeSusp_D_Stat>"

== system test_mdl_NI/To_NI_HIL/DSMC/DrvStatMonData ==
  in : Inport
  DrvEngLvlConfid_D_Stat : Subsystem
  DrvEngageLevel_No_Cnt : Subsystem
  DrvEngageLevel_No_Cs : Subsystem
  bus_creator : BusCreator  Inputs=3
  bus_selector : BusSelector  OutputSignals=DrvEngLvlConfid_D_Stat,DrvEngageLevel_No_Cs,DrvEngageLevel_No_Cnt
  out_port : Outport
  wires:
  bus_creator/1 -> out_port/1  "DrvStatMonData"
  DrvEngLvlConfid_D_Stat/1(out) -> bus_creator/1  "DrvEngLvlConfid_D_Stat"
  DrvEngageLevel_No_Cs/1(out) -> bus_creator/2  "DrvEngageLevel_No_Cs"
  DrvEngageLevel_No_Cnt/1(out) -> bus_creator/3  "DrvEngageLevel_No_Cnt"
  bus_selector/1 -> DrvEngLvlConfid_D_Stat/1(in)  "<DrvEngLvlConfid_D_Stat>"
  bus_selector/2 -> DrvEngageLevel_No_Cs/1(in)  "<DrvEngageLevel_No_Cs>"
  bus_selector/3 -> DrvEngageLevel_No_Cnt/1(in)  "<DrvEngageLevel_No_Cnt>"
  in/1 -> bus_selector/1

== system test_mdl_NI/To_NI_HIL/MRR/CAN_DET_AZIMUTH_01[rad] ==
  in : Inport
  out : Outport
  wires:
  in/1 -> out/1

== system test_mdl_NI/To_NI_HIL/MRR/CAN_DET_AZIMUTH_02[rad] ==
  in : Inport
  out : Outport
  wires:
  in/1 -> out/1

== system test_mdl_NI/To_NI_HIL/MRR/CAN_DET_AZIMUTH_03[rad] ==
  in : Inport
  out : Outport
  wires:
  in/1 -> out/1

== system test_mdl_NI/To_NI_HIL/MRR/CAN_DET_ELEVATION_01[rad] ==
  in : Inport
  out : Outport
  wires:
  in/1 -> out/1

== system test_mdl_NI/To_NI_HIL/MRR/CAN_DET_ELEVATION_02[rad] ==
  in : Inport
  out : Outport
  wires:
  in/1 -> out/1

== system test_mdl_NI/To_NI_HIL/MRR/CAN_DET_ELEVATION_03[rad] ==
  in : Inport
  out : Outport
  wires:
  in/1 -> out/1

== system test_mdl_NI/To_NI_HIL/MRR/CAN_DET_RANGE_01[m] ==
  in : Inport
  out : Outport
  wires:
  in/1 -> out/1

== system test_mdl_NI/To_NI_HIL/MRR/CAN_DET_RANGE_02[m] ==
  in : Inport
  out : Outport
  wires:
  in/1 -> out/1

== system test_mdl_NI/To_NI_HIL/MRR/CAN_DET_RANGE_03[m] ==
  in : Inport
  out : Outport
  wires:
  in/1 -> out/1

== system test_mdl_NI/To_NI_HIL/MRR/CAN_DET_RANGE_RATE_01[m|s] ==
  in : Inport
  out : Outport
  wires:
  in/1 -> out/1

== system test_mdl_NI/To_NI_HIL/MRR/CAN_DET_RANGE_RATE_02[m|s] ==
  in : Inport
  out : Outport
  wires:
  in/1 -> out/1

== system test_mdl_NI/To_NI_HIL/MRR/CAN_DET_RANGE_RATE_03[m|s] ==
  in : Inport
  out : Outport
  wires:
  in/1 -> out/1

== system test_mdl_NI/To_NI_HIL/SRR_L/FL_SOD ==
  in : Inport
  SRR_FL_001 : Subsystem
  SRR_FL_002 : Subsystem
  SRR_FL_003 : Subsystem
  bus_creator : BusCreator  Inputs=3
  bus_selector : BusSelector  OutputSignals=SRR_FL_001,SRR_FL_002,SRR_FL_003
  out_port : Outport
  wires:
  bus_creator/1 -> out_port/1  "FL_SOD"
  SRR_FL_001/1(out_port) -> bus_creator/1  "SRR_FL_001"
  SRR_FL_002/1(out_port) -> bus_creator/2  "SRR_FL_002"
  SRR_FL_003/1(out_port) -> bus_creator/3  "SRR_FL_003"
  bus_selector/1 -> SRR_FL_001/1(in)  "<SRR_FL_001>"
  bus_selector/2 -> SRR_FL_002/1(in)  "<SRR_FL_002>"
  bus_selector/3 -> SRR_FL_003/1(in)  "<SRR_FL_003>"
  in/1 -> bus_selector/1

== system test_mdl_NI/To_NI_HIL/SRR_L/RL_SOD ==
  in : Inport
  SRR_RL_001 : Subsystem
  SRR_RL_002 : Subsystem
  SRR_RL_003 : Subsystem
  bus_creator : BusCreator  Inputs=3
  bus_selector : BusSelector  OutputSignals=SRR_RL_001,SRR_RL_002,SRR_RL_003
  out_port : Outport
  wires:
  bus_creator/1 -> out_port/1  "RL_SOD"
  SRR_RL_001/1(out_port) -> bus_creator/1  "SRR_RL_001"
  SRR_RL_002/1(out_port) -> bus_creator/2  "SRR_RL_002"
  SRR_RL_003/1(out_port) -> bus_creator/3  "SRR_RL_003"
  bus_selector/1 -> SRR_RL_001/1(in)  "<SRR_RL_001>"
  bus_selector/2 -> SRR_RL_002/1(in)  "<SRR_RL_002>"
  bus_selector/3 -> SRR_RL_003/1(in)  "<SRR_RL_003>"
  in/1 -> bus_selector/1

== system test_mdl_NI/To_NI_HIL/SRR_R/FR_SOD ==
  in : Inport
  SRR_FR_001 : Subsystem
  SRR_FR_002 : Subsystem
  SRR_FR_003 : Subsystem
  bus_creator : BusCreator  Inputs=3
  bus_selector : BusSelector  OutputSignals=SRR_FR_001,SRR_FR_002,SRR_FR_003
  out_port : Outport
  wires:
  bus_creator/1 -> out_port/1  "FR_SOD"
  SRR_FR_001/1(out_port) -> bus_creator/1  "SRR_FR_001"
  SRR_FR_002/1(out_port) -> bus_creator/2  "SRR_FR_002"
  SRR_FR_003/1(out_port) -> bus_creator/3  "SRR_FR_003"
  bus_selector/1 -> SRR_FR_001/1(in)  "<SRR_FR_001>"
  bus_selector/2 -> SRR_FR_002/1(in)  "<SRR_FR_002>"
  bus_selector/3 -> SRR_FR_003/1(in)  "<SRR_FR_003>"
  in/1 -> bus_selector/1

== system test_mdl_NI/To_NI_HIL/SRR_R/RR_SOD ==
  in : Inport
  SRR_RR_001 : Subsystem
  SRR_RR_002 : Subsystem
  SRR_RR_003 : Subsystem
  bus_creator : BusCreator  Inputs=3
  bus_selector : BusSelector  OutputSignals=SRR_RR_001,SRR_RR_002,SRR_RR_003
  out_port : Outport
  wires:
  bus_creator/1 -> out_port/1  "RR_SOD"
  SRR_RR_001/1(out_port) -> bus_creator/1  "SRR_RR_001"
  SRR_RR_002/1(out_port) -> bus_creator/2  "SRR_RR_002"
  SRR_RR_003/1(out_port) -> bus_creator/3  "SRR_RR_003"
  bus_selector/1 -> SRR_RR_001/1(in)  "<SRR_RR_001>"
  bus_selector/2 -> SRR_RR_002/1(in)  "<SRR_RR_002>"
  bus_selector/3 -> SRR_RR_003/1(in)  "<SRR_RR_003>"
  in/1 -> bus_selector/1

== system test_mdl_NI/To_NI_HIL/Soft_ABS/ABS_BrkBst_Data ==
  in : Inport
  BrkTotTqRqDrv_No_Cnt : Subsystem
  BrkTotTqRqDrv_No_Cs : Subsystem
  BrkTot_Tq_RqDrv : Subsystem
  bus_creator : BusCreator  Inputs=3
  bus_selector : BusSelector  OutputSignals=BrkTot_Tq_RqDrv,BrkTotTqRqDrv_No_Cs,BrkTotTqRqDrv_No_Cnt
  out_port : Outport
  wires:
  bus_creator/1 -> out_port/1  "ABS_BrkBst_Data"
  BrkTot_Tq_RqDrv/1(out) -> bus_creator/1  "BrkTot_Tq_RqDrv"
  BrkTotTqRqDrv_No_Cs/1(out) -> bus_creator/2  "BrkTotTqRqDrv_No_Cs"
  BrkTotTqRqDrv_No_Cnt/1(out) -> bus_creator/3  "BrkTotTqRqDrv_No_Cnt"
  bus_selector/1 -> BrkTot_Tq_RqDrv/1(in)  "<BrkTot_Tq_RqDrv>"
  bus_selector/2 -> BrkTotTqRqDrv_No_Cs/1(in)  "<BrkTotTqRqDrv_No_Cs>"
  bus_selector/3 -> BrkTotTqRqDrv_No_Cnt/1(in)  "<BrkTotTqRqDrv_No_Cnt>"
  in/1 -> bus_selector/1

== system test_mdl_NI/To_NI_HIL/Soft_ABS/Accel_Data ==
  in : Inport
  VehLat2_A_Actl : Subsystem
  VehLong2_A_Actl : Subsystem
  bus_creator : BusCreator  Inputs=2
  bus_selector : BusSelector  OutputSignals=VehLong2_A_Actl,VehLat2_A_Actl
  out_port : Outport
  wires:
  bus_creator/1 -> out_port/1  "Accel_Data"
  VehLong2_A_Actl/1(out) -> bus_creator/1  "VehLong2_A_Actl"
  VehLat2_A_Actl/1(out) -> bus_creator/2  "VehLat2_A_Actl"
  bus_selector/1 -> VehLong2_A_Actl/1(in)  "<VehLong2_A_Actl>"
  bus_selector/2 -> VehLat2_A_Actl/1(in)  "<VehLat2_A_Actl>"
  in/1 -> bus_selector/1

== system test_mdl_NI/To_NI_HIL/Soft_ABS/BrakeSnData_3 ==
  in : Inport
  VehLatComp_A_Actl : Subsystem
  VehLongComp_A_Actl : Subsystem
  VehOverGnd_V_Est : Subsystem
  VehYawComp_W_Actl : Subsystem
  bus_creator : BusCreator  Inputs=4
  bus_selector : BusSelector  OutputSignals=VehYawComp_W_Actl,VehOverGnd_V_Est,VehLongComp_A_Actl,VehLatComp_A_Actl
  out_port : Outport
  wires:
  bus_creator/1 -> out_port/1  "BrakeSnData_3"
  VehYawComp_W_Actl/1(out) -> bus_creator/1  "VehYawComp_W_Actl"
  VehOverGnd_V_Est/1(out) -> bus_creator/2  "VehOverGnd_V_Est"
  VehLongComp_A_Actl/1(out) -> bus_creator/3  "VehLongComp_A_Actl"
  VehLatComp_A_Actl/1(out) -> bus_creator/4  "VehLatComp_A_Actl"
  bus_selector/1 -> VehYawComp_W_Actl/1(in)  "<VehYawComp_W_Actl>"
  bus_selector/2 -> VehOverGnd_V_Est/1(in)  "<VehOverGnd_V_Est>"
  bus_selector/3 -> VehLongComp_A_Actl/1(in)  "<VehLongComp_A_Actl>"
  bus_selector/4 -> VehLatComp_A_Actl/1(in)  "<VehLatComp_A_Actl>"
  in/1 -> bus_selector/1

== system test_mdl_NI/To_NI_HIL/Soft_ABS/BrakeSnData_4 ==
  in : Inport
  BrkTot_Tq_Actl : Subsystem
  VehRolComp_W_Actl : Subsystem
  VehVertComp_A_Actl : Subsystem
  bus_creator : BusCreator  Inputs=3
  bus_selector : BusSelector  OutputSignals=VehVertComp_A_Actl,VehRolComp_W_Actl,BrkTot_Tq_Actl
  out_port : Outport
  wires:
  bus_creator/1 -> out_port/1  "BrakeSnData_4"
  VehVertComp_A_Actl/1(out) -> bus_creator/1  "VehVertComp_A_Actl"
  VehRolComp_W_Actl/1(out) -> bus_creator/2  "VehRolComp_W_Actl"
  BrkTot_Tq_Actl/1(out) -> bus_creator/3  "BrkTot_Tq_Actl"
  bus_selector/1 -> VehVertComp_A_Actl/1(in)  "<VehVertComp_A_Actl>"
  bus_selector/2 -> VehRolComp_W_Actl/1(in)  "<VehRolComp_W_Actl>"
  bus_selector/3 -> BrkTot_Tq_Actl/1(in)  "<BrkTot_Tq_Actl>"
  in/1 -> bus_selector/1

== system test_mdl_NI/To_NI_HIL/Soft_ABS/BrakeSnData_5 ==
  in : Inport
  SteWhlComp_An_Est : Subsystem
  bus_creator : BusCreator  Inputs=1
  bus_selector : BusSelector  OutputSignals=SteWhlComp_An_Est
  out_port : Outport
  wires:
  bus_creator/1 -> out_port/1  "BrakeSnData_5"
  SteWhlComp_An_Est/1(out) -> bus_creator/1  "SteWhlComp_An_Est"
  bus_selector/1 -> SteWhlComp_An_Est/1(in)  "<SteWhlComp_An_Est>"
  in/1 -> bus_selector/1

== system test_mdl_NI/To_NI_HIL/Soft_ABS/BrakeSysFeatures ==
  in : Inport
  VehVActlBrk_No_Cnt : Subsystem
  VehVActlBrk_No_Cs : Subsystem
  Veh_V_ActlBrk : Subsystem
  bus_creator : BusCreator  Inputs=3
  bus_selector : BusSelector  OutputSignals=Veh_V_ActlBrk,VehVActlBrk_No_Cs,VehVActlBrk_No_Cnt
  out_port : Outport
  wires:
  bus_creator/1 -> out_port/1  "BrakeSysFeatures"
  Veh_V_ActlBrk/1(out) -> bus_creator/1  "Veh_V_ActlBrk"
  VehVActlBrk_No_Cs/1(out) -> bus_creator/2  "VehVActlBrk_No_Cs"
  VehVActlBrk_No_Cnt/1(out) -> bus_creator/3  "VehVActlBrk_No_Cnt"
  bus_selector/1 -> Veh_V_ActlBrk/1(in)  "<Veh_V_ActlBrk>"
  bus_selector/2 -> VehVActlBrk_No_Cs/1(in)  "<VehVActlBrk_No_Cs>"
  bus_selector/3 -> VehVActlBrk_No_Cnt/1(in)  "<VehVActlBrk_No_Cnt>"
  in/1 -> bus_selector/1

== system test_mdl_NI/To_NI_HIL/Soft_ABS/BrakeSysFeatures_2 ==
  in : Inport
  BpedMove_D_Actl : Subsystem
  BpedMove_No_Cnt : Subsystem
  BpedMove_No_Cs : Subsystem
  bus_creator : BusCreator  Inputs=3
  bus_selector : BusSelector  OutputSignals=BpedMove_D_Actl,BpedMove_No_Cs,BpedMove_No_Cnt
  out_port : Outport
  wires:
  bus_creator/1 -> out_port/1  "BrakeSysFeatures_2"
  BpedMove_D_Actl/1(out) -> bus_creator/1  "BpedMove_D_Actl"
  BpedMove_No_Cs/1(out) -> bus_creator/2  "BpedMove_No_Cs"
  BpedMove_No_Cnt/1(out) -> bus_creator/3  "BpedMove_No_Cnt"
  bus_selector/1 -> BpedMove_D_Actl/1(in)  "<BpedMove_D_Actl>"
  bus_selector/2 -> BpedMove_No_Cs/1(in)  "<BpedMove_No_Cs>"
  bus_selector/3 -> BpedMove_No_Cnt/1(in)  "<BpedMove_No_Cnt>"
  in/1 -> bus_selector/1

== system test_mdl_NI/To_NI_HIL/Soft_ABS/DesiredTorqBrk ==
  in : Inport
  AccBrkActv_B_Actl : Subsystem
  AccBrkPrchgActv_B_Actl : Subsystem
  AccBrkTotTqMn_B_Actl : Subsystem
  AccStopActv_B_ActlBrk : Subsystem
  CmbbBaSensInc_B_Actl : Subsystem
  CmbbBrkDecel_B_Actl : Subsystem
  CmbbBrkPrchg_B_Actl : Subsystem
  VehLongOvrGnd_A_Est : Subsystem
  VehStop_D_Stat : Subsystem
  VehicleStationary : Subsystem
  bus_creator : BusCreator  Inputs=10
  bus_selector : BusSelector  OutputSignals=AccBrkPrchgActv_B_Actl,AccBrkActv_B_Actl,AccStopActv_B_ActlBrk,CmbbBrkPrchg_B_Actl,CmbbBaSensInc_B_Actl,CmbbBrkDecel_B_Actl,VehicleStationary,VehStop_D_Stat,VehLongOvrGnd_A_Est,AccBrkTotTqMn_B_Actl
  out_port : Outport
  wires:
  bus_creator/1 -> out_port/1  "DesiredTorqBrk"
  AccBrkPrchgActv_B_Actl/1(out) -> bus_creator/1  "AccBrkPrchgActv_B_Actl"
  AccBrkActv_B_Actl/1(out) -> bus_creator/2  "AccBrkActv_B_Actl"
  AccStopActv_B_ActlBrk/1(out) -> bus_creator/3  "AccStopActv_B_ActlBrk"
  CmbbBrkPrchg_B_Actl/1(out) -> bus_creator/4  "CmbbBrkPrchg_B_Actl"
  CmbbBaSensInc_B_Actl/1(out) -> bus_creator/5  "CmbbBaSensInc_B_Actl"
  CmbbBrkDecel_B_Actl/1(out) -> bus_creator/6  "CmbbBrkDecel_B_Actl"
  VehicleStationary/1(out) -> bus_creator/7  "VehicleStationary"
  VehStop_D_Stat/1(out) -> bus_creator/8  "VehStop_D_Stat"
  VehLongOvrGnd_A_Est/1(out) -> bus_creator/9  "VehLongOvrGnd_A_Est"
  AccBrkTotTqMn_B_Actl/1(out) -> bus_creator/10  "AccBrkTotTqMn_B_Actl"
  bus_selector/1 -> AccBrkPrchgActv_B_Actl/1(in)  "<AccBrkPrchgActv_B_Actl>"
  bus_selector/2 -> AccBrkActv_B_Actl/1(in)  "<AccBrkActv_B_Actl>"
  bus_selector/3 -> AccStopActv_B_ActlBrk/1(in)  "<AccStopActv_B_ActlBrk>"
  bus_selector/4 -> CmbbBrkPrchg_B_Actl/1(in)  "<CmbbBrkPrchg_B_Actl>"
  bus_selector/5 -> CmbbBaSensInc_B_Actl/1(in)  "<CmbbBaSensInc_B_Actl>"
  bus_selector/6 -> CmbbBrkDecel_B_Actl/1(in)  "<CmbbBrkDecel_B_Actl>"
  bus_selector/7 -> VehicleStationary/1(in)  "<VehicleStationary>"
  bus_selector/8 -> VehStop_D_Stat/1(in)  "<VehStop_D_Stat>"
  bus_selector/9 -> VehLongOvrGnd_A_Est/1(in)  "<VehLongOvrGnd_A_Est>"
  bus_selector/10 -> AccBrkTotTqMn_B_Actl/1(in)  "<AccBrkTotTqMn_B_Actl>"
  in/1 -> bus_selector/1

== system test_mdl_NI/To_NI_HIL/Soft_ABS/ToCarSim ==
  in : Inport
  MCPressure : Subsystem
  bus_creator : BusCreator  Inputs=1
  bus_selector : BusSelector  OutputSignals=MCPressure
  out_port : Outport
  wires:
  bus_creator/1 -> out_port/1  "ToCarSim"
  MCPressure/1(out) -> bus_creator/1  "MCPressure"
  bus_selector/1 -> MCPressure/1(in)  "<MCPressure>"
  in/1 -> bus_selector/1

== system test_mdl_NI/To_NI_HIL/Soft_ABS/WheelData ==
  in : Inport
  WhlDirRl_D_Actl : Subsystem
  WhlDirRr_D_Actl : Subsystem
  bus_creator : BusCreator  Inputs=2
  bus_selector : BusSelector  OutputSignals=WhlDirRl_D_Actl,WhlDirRr_D_Actl
  out_port : Outport
  wires:
  bus_creator/1 -> out_port/1  "WheelData"
  WhlDirRl_D_Actl/1(out) -> bus_creator/1  "WhlDirRl_D_Actl"
  WhlDirRr_D_Actl/1(out) -> bus_creator/2  "WhlDirRr_D_Actl"
  bus_selector/1 -> WhlDirRl_D_Actl/1(in)  "<WhlDirRl_D_Actl>"
  bus_selector/2 -> WhlDirRr_D_Actl/1(in)  "<WhlDirRr_D_Actl>"
  in/1 -> bus_selector/1
